simulink model "lanedetection"  (R2013b)
settings: Solver=FixedStepDiscrete  StartTime=0.0  StopTime=inf  RelTol=1e-3
libraries: embdlinuxlib x8
settings Model: SimulationMode=external  ExtModeTrigDuration=100  Creator=asus  LastModifiedBy=asus
settings OptimizationCC: OptimizeModelRefInitCode=on  LifeSpan=1
settings DebuggingCC: SolverPrmCheckMsg=none
settings HardwareCC: ProdLargestAtomicInteger=Long  ProdLargestAtomicFloat=Double  ProdEndianess=LittleEndian  ProdHWDeviceType=ARM Compatible->ARM Cortex
settings RTWCC: SystemTargetFile=realtime.tlc  GenerateMakefile=off  TemplateMakefile=realtime.tmf  Description=Run on Target Hardware  RTWVerbose=off  ProcessScript=realtime_make_rtw_hook
settings STFCustomTargetCC: TargetLibSuffix=.a  GenerateSampleERTMain=on  ERTCustomFileBanners=on  SupportNonInlinedSFcns=off  SupportVariableSizeSignals=on  MATLABClassNameForMDSCustomization=Simulink.SoftwareTarget.ERTCustomization  GRTInterface=off  SystemTargetFile=realtime.tlc
settings ERTTargetCC: CodeReplacementLibrary=ANSI_C  GenerateSampleERTMain=on  ParMdlRefBuildCompliant=off  CompOptLevelCompliant=off  ConcurrentExecutionCompliant=off  CombineOutputUpdateFcns=off  ERTFirstTimeCompliant=off  SupportContinuousTime=on  SupportVariableSizeSignals=on  ModelStepFunctionPrototypeControlCompliant=off  CPPClassGenCompliant=off  ExtMode=on  ExtModeMexArgs='169.254.0.2' 0 17725  InlinedParameterPlacement=NonHierarchical  ERTSrcFileBannerTemplate=realtime_code_template.cgt  ERTHdrFileBannerTemplate=realtime_code_template.cgt  ERTDataSrcFileTemplate=realtime_code_template.cgt  ERTDataHdrFileTemplate=realtime_code_template.cgt  ERTCustomFileTemplate=realtime_file_process.tlc

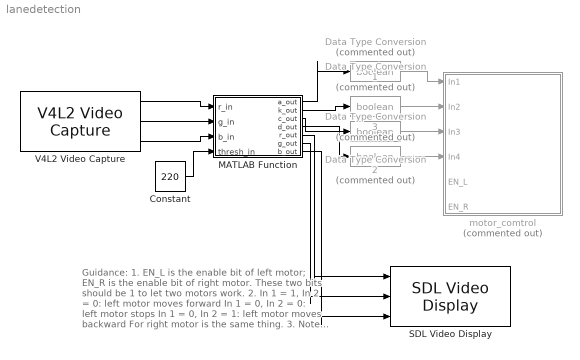
== system lanedetection ==
  note: Guidance:
      | 1. EN_L is the enable bit of left motor;
      | EN_R is the enable bit of right motor. These
      | two bits should be 1 to let two motors work.
      | 2. In 1 = 1, In 2 = 0: left motor moves forward
      |     In 1 = 0, In 2 = 0: left motor stops
      |     In 1 = 0, In 2 = 1: left motor moves backward
      |     For right motor is the same thing.
      | 3. Note that all the inputs type should be boolean.
  Constant : Constant  Value=220
  Data Type Conversion{,1..3} (4 alike) : DataTypeConversion  Commented=on  OutDataTypeStr=boolean
  MATLAB Function : MATLAB Function  TreatAsAtomicUnit=on
  SDL Video Display : embdlinuxlib/SDL Video Display  pixelFormat=RGB  pixelOrder=Planar  rowMajor=on  blockPlatform=Raspberry Pi
  V4L2 Video Capture : embdlinuxlib/V4L2 Video Capture  m_devName='/dev/video0'  roi=[0, 0, 640, 480]  imSizeSelection=320x240  imSize=[640, 480]  pixelFormat=RGB  pixelOrder=Planar  sampleTime=1/10  simOutput=Colorbars  blockPlatform=Raspberry Pi
  motor_comtrol : Subsystem  Commented=on
  wires:
  V4L2 Video Capture/1 -> MATLAB Function/1(r_in)
  V4L2 Video Capture/2 -> MATLAB Function/2(g_in)
  V4L2 Video Capture/3 -> MATLAB Function/3(b_in)
  Constant/1 -> MATLAB Function/4(thresh_in)
  MATLAB Function/1(a_out) -> Data Type Conversion/1
  MATLAB Function/2(k_out) -> Data Type Conversion1/1
  MATLAB Function/3(c_out) -> Data Type Conversion2/1
  MATLAB Function/4(d_out) -> Data Type Conversion3/1
  Data Type Conversion/1 -> motor_comtrol/1(In1)
  Data Type Conversion1/1 -> motor_comtrol/2(In2)
  Data Type Conversion2/1 -> motor_comtrol/3(In3)
  Data Type Conversion3/1 -> motor_comtrol/4(In4)
  MATLAB Function/5(r_out) -> SDL Video Display/1
  MATLAB Function/6(g_out) -> SDL Video Display/2
  MATLAB Function/7(b_out) -> SDL Video Display/3

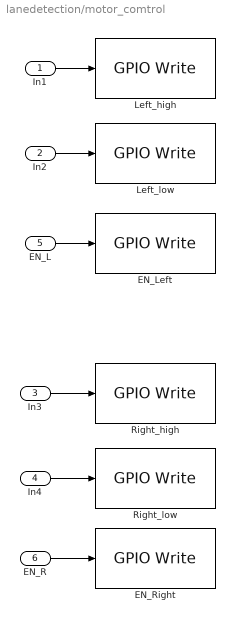
== system lanedetection/motor_comtrol ==
  In1 : Inport
  In2 : Inport  Port=2
  In3 : Inport  Port=3
  In4 : Inport  Port=4
  EN_L : Inport  Port=5
  EN_R : Inport  Port=6
  EN_Left : embdlinuxlib/GPIO Write  board=Model B Rev2  gpio=27  direction=Output  blockPlatform=Raspberry Pi
  EN_Right : embdlinuxlib/GPIO Write  board=Model B Rev2  gpio=22  direction=Output  blockPlatform=Raspberry Pi
  Left_high : embdlinuxlib/GPIO Write  board=Model B Rev2  gpio=4  direction=Output  blockPlatform=Raspberry Pi
  Left_low : embdlinuxlib/GPIO Write  board=Model B Rev2  gpio=17  direction=Output  blockPlatform=Raspberry Pi
  Right_high : embdlinuxlib/GPIO Write  board=Model B Rev2  gpio=23  direction=Output  blockPlatform=Raspberry Pi
  Right_low : embdlinuxlib/GPIO Write  board=Model B Rev2  gpio=24  direction=Output  blockPlatform=Raspberry Pi
  wires:
  EN_R/1 -> EN_Right/1
  EN_L/1 -> EN_Left/1
  In4/1 -> Right_low/1
  In2/1 -> Left_low/1
  In3/1 -> Right_high/1
  In1/1 -> Left_high/1

== matlab function lanedetection/MATLAB Function ==
  data: r_in input; a_out output; k_out output; g_in input; b_in input; c_out output; thresh_in input; d_out output; r_out output; g_out output; b_out output
function [a_out,k_out,c_out,d_out,r_out,g_out,b_out]=trackball(r_in,g_in,b_in,thresh_in)
%#codegen
r=r_in;
g=g_in;
b=b_in;
thresh=thresh_in;
nGray=0.299*r+0.587*g+0.114*b;
bw=nGray>thresh;
[x,y]=find(bw);
xm=mean(x);
ym=mean(y);
xx=max(1,xm-5):min(xm+5,size(bw,1));
yy=max(1,ym-5):min(ym+5,size(bw,2));
bwbw=zeros(size(bw),'uint8');
bwbw(xx,yy)=255;
r_out=uint8((r_in+bwbw));
g_out=uint8((g_in-bwbw));
b_out=uint8((b_in-bwbw));
if xm<110
    a_out=1;
    k_out=1;
    c_out=1;
    d_out=0;
elseif xm>210
    a_out=1;
    k_out=0;
    c_out=1;
    d_out=1;
    else
    a_out=1;
    k_out=0;
    c_out=1;
    d_out=0;
end
